simulink model "chap9_3sim"  (Simulink 8.1)
settings: Solver=ode45  StartTime=0.0  StopTime=10.0  RelTol=1e-3
settings Model: Creator=liujk  LastModifiedBy=liujk
settings DataIOCC: SignalLoggingName=sigsOut
settings OptimizationCC: ExpressionDepthLimit=128
settings DebuggingCC: SaveWithParameterizedLinksMsg=none  SignalResolutionControl=TryResolveAllWithWarning  SolverPrmCheckMsg=none  MultiTaskDSMMsg=warning  MultiTaskCondExecSysMsg=none  StrictBusMsg=None
settings HardwareCC: TargetUnknown=on
settings RTWCC: IncludeERTFirstTime=on

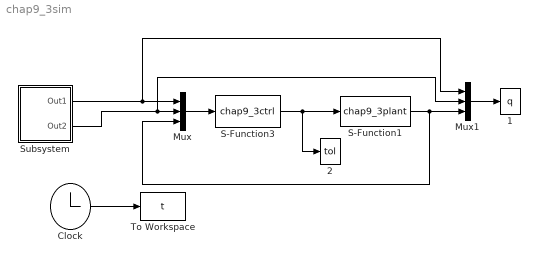
== system chap9_3sim ==
  "  1" : ToWorkspace  VariableName=q  SampleTime=-1
  "  2" : ToWorkspace  VariableName=tol  SampleTime=-1
  Clock : Clock
  Mux : Mux  Inputs=3
  Mux1 : Mux  Inputs=3
  S-Function1 : S-Function  FunctionName=chap9_3plant  EnableBusSupport=off
  S-Function3 : S-Function  FunctionName=chap9_3ctrl  EnableBusSupport=off
  Subsystem : Subsystem
  To Workspace : ToWorkspace  VariableName=t  SampleTime=-1
  wires:
  Clock/1 -> To Workspace/1
  S-Function3/1 -> "  2"/1, S-Function1/1
  Mux/1 -> S-Function3/1
  S-Function1/1 -> Mux1/3, Mux/3
  Mux1/1 -> "  1"/1
  Subsystem/1(Out1) -> Mux1/1, Mux/1
  Subsystem/2(Out2) -> Mux1/2, Mux/2

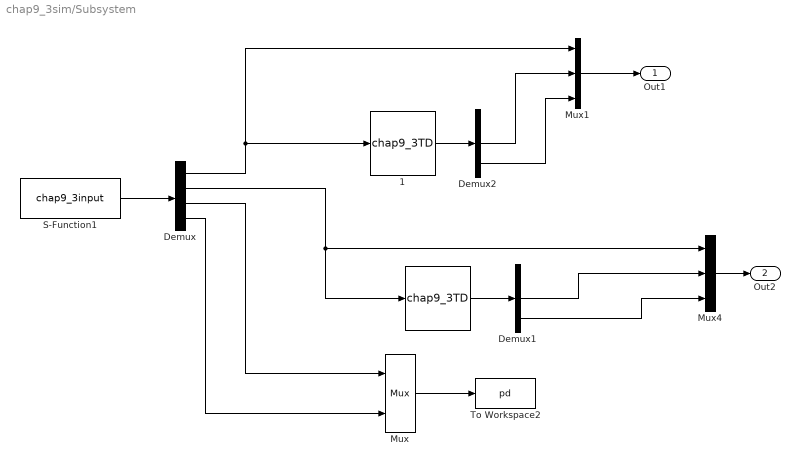
== system chap9_3sim/Subsystem ==
  " " : S-Function  FunctionName=chap9_3TD  EnableBusSupport=off
  " 1" : S-Function  FunctionName=chap9_3TD  EnableBusSupport=off
  Demux : Demux
  Demux1 : Demux  Outputs=3
  Demux2 : Demux  Outputs=3
  Mux : Mux  Inputs=2
  Mux1 : Mux  Inputs=3
  Mux4 : Mux  Inputs=3
  S-Function1 : S-Function  FunctionName=chap9_3input  EnableBusSupport=off
  To Workspace2 : ToWorkspace  VariableName=pd  SampleTime=-1
  Out1 : Outport
  Out2 : Outport  Port=2
  wires:
  S-Function1/1 -> Demux/1
  Demux2/3 -> Mux1/3
  Mux1/1 -> Out1/1
  Mux4/1 -> Out2/1
  Demux/1 -> " 1"/1, Mux1/1
  Demux/2 -> " "/1, Mux4/1
  Demux/3 -> Mux/1
  Demux/4 -> Mux/2
  Mux/1 -> To Workspace2/1
  " "/1 -> Demux1/1
  Demux1/2 -> Mux4/2
  Demux1/3 -> Mux4/3
  " 1"/1 -> Demux2/1
  Demux2/2 -> Mux1/2
